simulink model "Doppelpendel_LQG_2014b"  (R2014b)
settings: Solver=ode45  StartTime=0.0  StopTime=15
values from neighbouring files (symbols this model uses):
  Beobachter_Rueckfuehrung = 1    [LoadParameter.m]
  Kalman_Filter = 2    [LoadParameter.m]
  parLQR = LQR_Entwurf(sysd,parLQR)    [A2_5.m]
  Quantisierung = 0    [LoadParameter.m]
undefined symbols (not defined in the file or in its folder): parDP, parKAL
libraries: cstblocks x3
settings Model: CovSFcnEnable=on  Creator=tg  LastModifiedBy=Daniel
settings DataIOCC: SignalLoggingSaveFormat=ModelDataLogs
settings OptimizationCC: ExpressionDepthLimit=2147483647  InitFltsAndDblsToZero=on
settings DebuggingCC: UnderspecifiedInitializationDetection=Classic  MergeDetectMultiDrivingBlocksExec=none  FcnCallInpInsideContextMsg=UseLocalSettings  FrameProcessingCompatibilityMsg=error  StateNameClashWarn=warning
settings SFSimCC: SimParseCustomCode=off
settings GRTTargetCC: CombineOutputUpdateFcns=off  GRTInterface=on

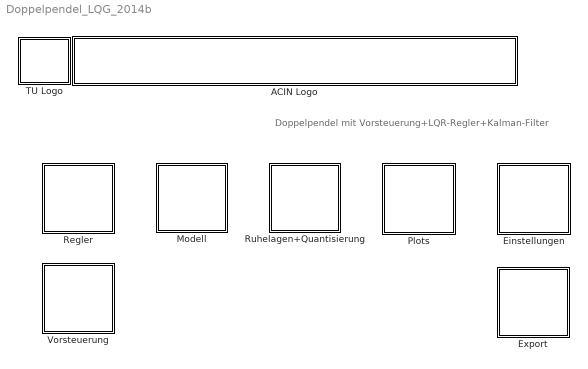
== system Doppelpendel_LQG_2014b ==
  note: Doppelpendel mit Vorsteuerung+LQR-Regler+Kalman-Filter
  ACIN Logo : Subsystem
      mask init:
      | s = get_param(gcb,'UserData');
      mask Display:
      | image(s.logo,[0 0 439 45]);
      | %axis image
  Einstellungen : Subsystem
  Export : Subsystem
  Modell : Subsystem
  Plots : Subsystem
  Regler : Subsystem
  Ruhelagen+Quantisierung : Subsystem
  TU Logo : Subsystem
      mask init:
      | s = get_param(gcb,'UserData');
      mask Display: image(s.logo,[0 0 45 45]);
  Vorsteuerung : Subsystem

== system Doppelpendel_LQG_2014b/ACIN Logo ==

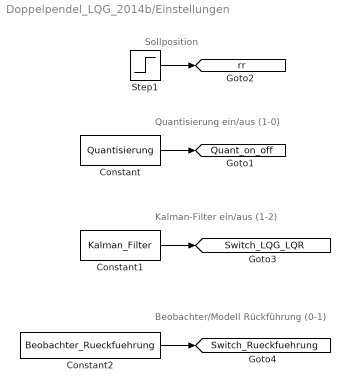
== system Doppelpendel_LQG_2014b/Einstellungen ==
  note: Sollposition
  note: Quantisierung ein/aus (1-0)
  note: Kalman-Filter ein/aus (1-2)
  note: Beobachter/Modell Rückführung (0-1)
  Constant : Constant  Value=Quantisierung
  Constant1 : Constant  Value=Kalman_Filter
  Constant2 : Constant  Value=Beobachter_Rueckfuehrung
  Step1 : Step  After=0.1  SampleTime=parLQR.Ta
  tag scope: Quant_on_off=global, Switch_LQG_LQR=global, Switch_Rueckfuehrung=global, rr=global
  wires:
  Step1/1 -> [rr]
  Constant/1 -> [Quant_on_off]
  Constant1/1 -> [Switch_LQG_LQR]
  Constant2/1 -> [Switch_Rueckfuehrung]

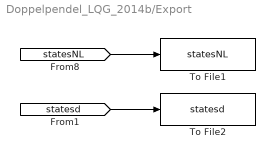
== system Doppelpendel_LQG_2014b/Export ==
  To File1 : ToFile  Filename=statesNL  MatrixName=data  SampleTime=parDP.Ta
  To File2 : ToFile  Filename=statesd  MatrixName=data  SampleTime=parDP.Ta
  wires:
  [statesNL] -> To File1/1
  [statesd] -> To File2/1

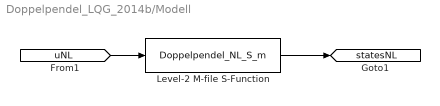
== system Doppelpendel_LQG_2014b/Modell ==
  Level-2 M-file S-Function : M-S-Function  FunctionName=Doppelpendel_NL_S_m  Parameters=parDP.phi10,parDP.omega10,parDP.phi20,parDP.omega20,parDP.s0,parDP.w0,parDP.l1,parDP.l2,parDP.a1,parDP.a2,parDP.m1,parDP.m2,parDP.J1,parDP.J2,parDP.d1,parDP.d2
  tag scope: statesNL=global
  wires:
  [uNL] -> Level-2 M-file S-Function/1
  Level-2 M-file S-Function/1 -> [statesNL]

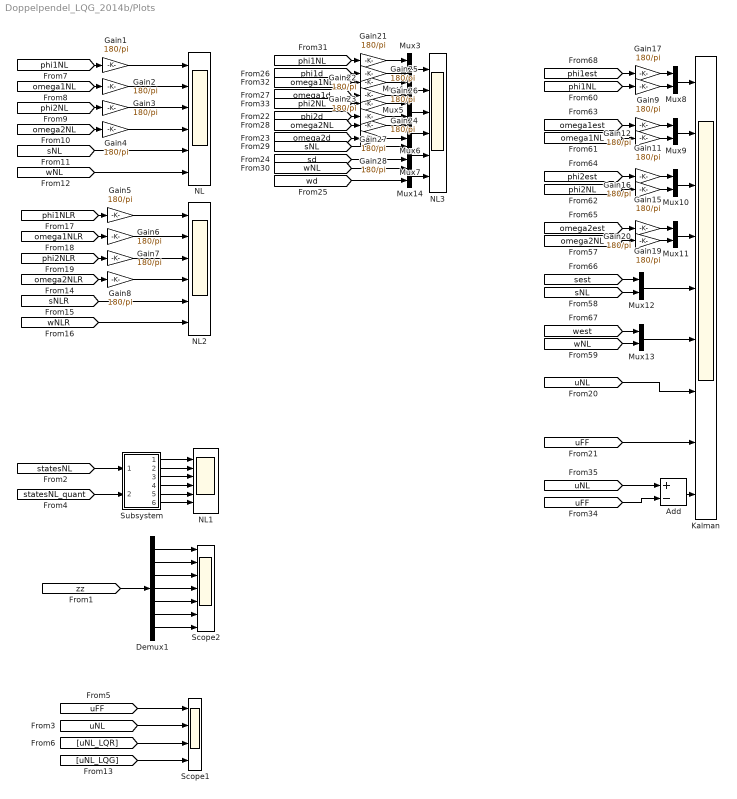
== system Doppelpendel_LQG_2014b/Plots ==
  Add : Sum  Inputs=+-
  Demux1 : Demux  Outputs=7
  Gain{1..9,11..12,15..17,19..28} (24 alike) : Gain  Gain=180/pi
  Kalman : Scope  NumInputPorts=9
      settings: TimeRange=auto  ShowLegends=on  MaxDataPoints=5000  SaveToWorkspace=off  SaveName=ScopeData6  YMin=176.91117~-10.79662~175.59226~-16.92479~-0.25002~-0.32868~-0.36253~-0.36233~-0.00149  YMax=183.0881~10.79663~184.40772~16.91023~0.25002~0.32868~0.36251~0.36233~0.0017  SampleTime=-1
  Mux{3..14} (12 alike) : Mux  Inputs=2
  NL{,1..3} (4 alike) : Scope  NumInputPorts=6
      NL settings: TimeRange=auto  MaxDataPoints=5000  SaveToWorkspace=off  SaveName=ScopeData2  YMin=175.44386~-8.63425~173.59154~-18.09348~-0.06241~-0.43407  YMax=186.73106~14.24878~186.84811~25.58372~0.56166~0.4085  SampleTime=-1
      NL1 settings: TimeRange=auto  MaxDataPoints=5000  SaveToWorkspace=off  YMin=-11.8659~-38.36034~-9.4516~-29.42~-0.73232~-1.57518  YMax=12.13115~31.29264~9.4588~20.36561~0.69417~0.92013  SampleTime=-1
      NL2 settings: TimeRange=auto  MaxDataPoints=5000  SaveToWorkspace=off  SaveName=ScopeData5  YMin=-11.8659~-37.01583~-9.4516~-28.16862~-0.73232~-1.55181  YMax=12.13115~30.14181~9.4588~19.57762~0.69415~0.90614  SampleTime=-1
      NL3 settings: TimeRange=6  MaxDataPoints=5000  SaveToWorkspace=off  SaveName=ScopeData8  YMin=-118.87207~-1672.77009~-161.23535~-3140.598~-141642.31686~-3281468.1161  YMax=19.55566~682.35836~19.81934~939.36059~15738.03521~364607.56846  SampleTime=-1
  Scope1 : Scope  NumInputPorts=4
      settings: TimeRange=6  MaxDataPoints=5000  SaveToWorkspace=off  SaveName=ScopeData4  YMin=-0.36233~-0.36253~-1.00000~-1.00000  YMax=0.36233~0.36251~1.00000~1.00000  SampleTime=-1
  Scope2 : Scope  NumInputPorts=7
      settings: TimeRange=6  MaxDataPoints=5000  SaveToWorkspace=off  SaveName=ScopeData9  YMin=-0.00026~-0.00051~-0.00077~-0.00273~-0.00865~-0.03633~-0.14821  YMax=0.00026~0.00051~0.00077~0.00273~0.00865~0.03633~0.14821  SampleTime=-1
  Subsystem : Subsystem
  wires:
  [omega1NL] -> Gain2/1
  [omega2NL] -> Gain4/1
  [sNL] -> NL/5
  [wNL] -> NL/6
  Gain1/1 -> NL/1
  Gain2/1 -> NL/2
  Gain3/1 -> NL/3
  Gain4/1 -> NL/4
  [phi1NL] -> Gain1/1
  [phi2NL] -> Gain3/1
  [statesNL] -> Subsystem/1(In1)
  [statesNL_quant] -> Subsystem/2(In2)
  Subsystem/1(Out1) -> NL1/1
  Subsystem/2(Out2) -> NL1/2
  Subsystem/3(Out3) -> NL1/3
  Subsystem/4(Out4) -> NL1/4
  Subsystem/5(Out5) -> NL1/5
  Subsystem/6(Out6) -> NL1/6
  [omega1NL] -> Gain22/1
  [omega2NL] -> Gain24/1
  [phi1NL] -> Gain21/1
  [phi2NL] -> Gain23/1
  Mux3/1 -> NL3/1
  Mux4/1 -> NL3/2
  Mux5/1 -> NL3/3
  Mux6/1 -> NL3/4
  Mux7/1 -> NL3/5
  Mux14/1 -> NL3/6
  Gain21/1 -> Mux3/1
  Gain22/1 -> Mux4/1
  Gain23/1 -> Mux5/1
  Gain24/1 -> Mux6/1
  [sNL] -> Mux7/1
  [wNL] -> Mux14/1
  [phi1d] -> Gain25/1
  [omega1d] -> Gain26/1
  [phi2d] -> Gain27/1
  [omega2d] -> Gain28/1
  Gain25/1 -> Mux3/2
  Gain26/1 -> Mux4/2
  Gain27/1 -> Mux5/2
  Gain28/1 -> Mux6/2
  [sd] -> Mux7/2
  [wd] -> Mux14/2
  Demux1/1 -> Scope2/1
  Demux1/2 -> Scope2/2
  Demux1/3 -> Scope2/3
  Demux1/4 -> Scope2/4
  Demux1/5 -> Scope2/5
  Demux1/6 -> Scope2/6
  Demux1/7 -> Scope2/7
  [zz] -> Demux1/1
  Mux13/1 -> Kalman/6
  Mux12/1 -> Kalman/5
  Mux11/1 -> Kalman/4
  [omega1NL] -> Gain12/1
  [omega2NL] -> Gain20/1
  [phi1NL] -> Gain9/1
  [phi2NL] -> Gain16/1
  [sest] -> Mux12/1
  [west] -> Mux13/1
  [sNL] -> Mux12/2
  [wNL] -> Mux13/2
  Gain9/1 -> Mux8/2
  Gain17/1 -> Mux8/1
  [phi1est] -> Gain17/1
  Mux8/1 -> Kalman/1
  Gain12/1 -> Mux9/2
  Gain11/1 -> Mux9/1
  Mux9/1 -> Kalman/2
  [omega1est] -> Gain11/1
  Gain16/1 -> Mux10/2
  Gain15/1 -> Mux10/1
  [phi2est] -> Gain15/1
  Mux10/1 -> Kalman/3
  Gain20/1 -> Mux11/2
  Gain19/1 -> Mux11/1
  [omega2est] -> Gain19/1
  [uFF] -> Scope1/1
  [uNL] -> Scope1/2
  [uNL_LQR] -> Scope1/3
  [uNL_LQG] -> Scope1/4
  [omega1NLR] -> Gain6/1
  [omega2NLR] -> Gain8/1
  [sNLR] -> NL2/5
  [wNLR] -> NL2/6
  Gain5/1 -> NL2/1
  Gain6/1 -> NL2/2
  Gain7/1 -> NL2/3
  Gain8/1 -> NL2/4
  [phi1NLR] -> Gain5/1
  [phi2NLR] -> Gain7/1
  [uNL] -> Kalman/7
  [uFF] -> Kalman/8
  Add/1 -> Kalman/9
  [uNL] -> Add/1
  [uFF] -> Add/2

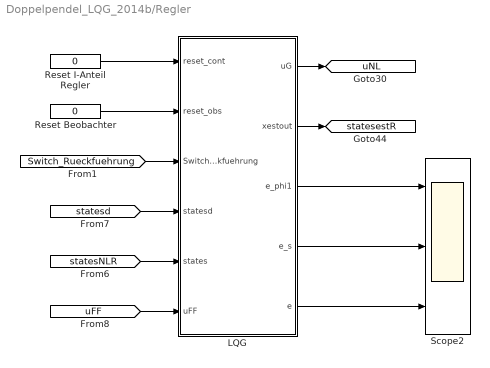
== system Doppelpendel_LQG_2014b/Regler ==
  LQG : MATLAB Function  TreatAsAtomicUnit=on
      settings: PermitHierarchicalResolution=ParametersOnly
  Reset Beobachter : Constant  Value=0
  Reset I-Anteil Regler : Constant  Value=0
  Scope2 : Scope  NumInputPorts=3
      settings: TimeRange=auto  MaxDataPoints=5000  SaveToWorkspace=off  SaveName=ScopeData  YMin=-0.00033~-0.00072~-30.14504  YMax=0.00036~0.00074~27.50332  SampleTime=-1
  tag scope: statesestR=global, uNL=global
  wires:
  LQG/3(e_phi1) -> Scope2/1
  LQG/4(e_s) -> Scope2/2
  LQG/5(e) -> Scope2/3
  [statesNLR] -> LQG/5(states)
  LQG/2(xestout) -> [statesestR]
  [statesd] -> LQG/4(statesd)
  [uFF] -> LQG/6(uFF)
  LQG/1(uG) -> [uNL]
  Reset Beobachter/1 -> LQG/2(reset_obs)
  Reset I-Anteil Regler/1 -> LQG/1(reset_cont)
  [Switch_Rueckfuehrung] -> LQG/3(Switch_Rueckfuehrung)

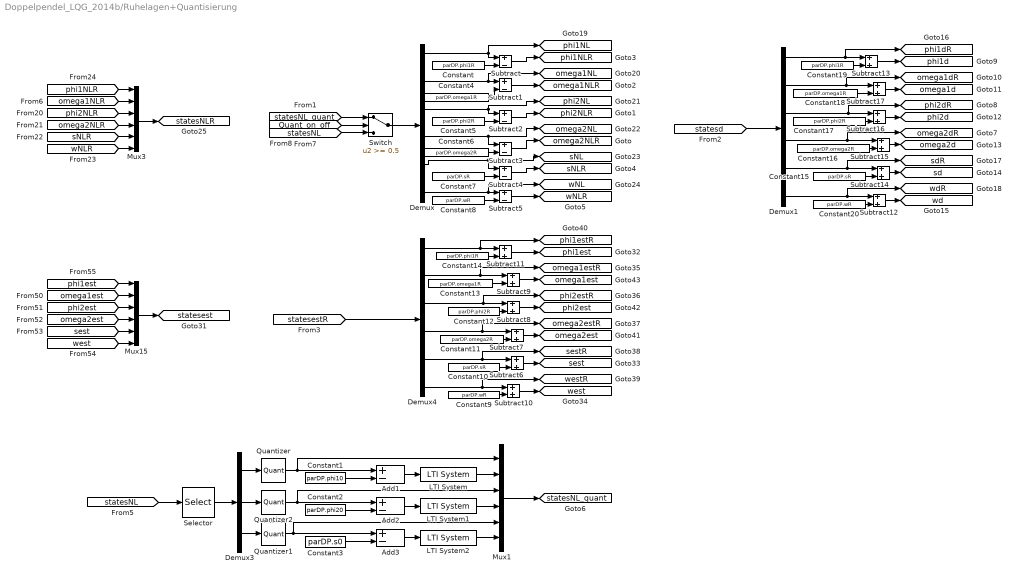
== system Doppelpendel_LQG_2014b/Ruhelagen+Quantisierung ==
  Add1 : Sum  Inputs=+-
  Add2 : Sum  Inputs=+-
  Add3 : Sum  Inputs=+-
  Constant : Constant  Value=parDP.phi1R
  Constant1 : Constant  Value=parDP.phi10
  Constant10 : Constant  Value=parDP.sR
  Constant11 : Constant  Value=parDP.omega2R
  Constant12 : Constant  Value=parDP.phi2R
  Constant13 : Constant  Value=parDP.omega1R
  Constant14 : Constant  Value=parDP.phi1R
  Constant15 : Constant  Value=parDP.sR
  Constant16 : Constant  Value=parDP.omega2R
  Constant17 : Constant  Value=parDP.phi2R
  Constant18 : Constant  Value=parDP.omega1R
  Constant19 : Constant  Value=parDP.phi1R
  Constant2 : Constant  Value=parDP.phi20
  Constant20 : Constant  Value=parDP.wR
  Constant3 : Constant  Value=parDP.s0
  Constant4 : Constant  Value=parDP.omega1R
  Constant5 : Constant  Value=parDP.phi2R
  Constant6 : Constant  Value=parDP.omega2R
  Constant7 : Constant  Value=parDP.sR
  Constant8 : Constant  Value=parDP.wR
  Constant9 : Constant  Value=parDP.wR
  Demux : Demux  Outputs=6
  Demux1 : Demux  Outputs=6
  Demux3 : Demux  Outputs=3
  Demux4 : Demux  Outputs=6
  LTI System : cstblocks/LTI System  sys=Fd_diff  IC=[]
  LTI System1 : cstblocks/LTI System  sys=Fd_diff  IC=[]
  LTI System2 : cstblocks/LTI System  sys=Fd_diff  IC=[]
  Mux1 : Mux  Inputs=6
  Mux15 : Mux  Inputs=6
  Mux3 : Mux  Inputs=6
  Quantizer : Quantizer  QuantizationInterval=Phiquantisierung  SampleTime=parLQR.Ta
  Quantizer1 : Quantizer  QuantizationInterval=Wegquantisierung  SampleTime=parLQR.Ta
  Quantizer2 : Quantizer  QuantizationInterval=Phiquantisierung  SampleTime=parLQR.Ta
  Selector : Selector  InputPortWidth=6  IndexOptions=Index vector (dialog)  Indices=[1 3 5]  OutputSizes=1
  Subtract{,1..5} (6 alike) : Sum  Inputs=+-
  Subtract{6..17} (12 alike) : Sum
  Switch : Switch  Threshold=0.5
  tag scope: omega1NL=global, omega1NLR=global, omega1d=global, omega1dR=global, omega1est=global, omega1estR=global, omega2NL=global, omega2NLR=global, omega2d=global, omega2dR=global, omega2est=global, omega2estR=global, phi1NL=global, phi1NLR=global, phi1d=global, phi1dR=global, phi1est=global, phi1estR=global, phi2NL=global, phi2NLR=global, phi2d=global, phi2dR=global, phi2est=global, phi2estR=global, sNL=global, sNLR=global, sd=global, sdR=global, sest=global, sestR=global, statesNLR=global, statesNL_quant=global, statesest=global, wNL=global, wNLR=global, wd=global, wdR=global, west=global, westR=global
  wires:
  [phi1NLR] -> Mux3/1
  [omega1NLR] -> Mux3/2
  [phi2NLR] -> Mux3/3
  [omega2NLR] -> Mux3/4
  [sNLR] -> Mux3/5
  [wNLR] -> Mux3/6
  Mux3/1 -> [statesNLR]
  [phi1est] -> Mux15/1
  [omega1est] -> Mux15/2
  [phi2est] -> Mux15/3
  [omega2est] -> Mux15/4
  [sest] -> Mux15/5
  [west] -> Mux15/6
  Mux15/1 -> [statesest]
  [statesNL] -> Selector/1
  Selector/1 -> Demux3/1
  Demux3/2 -> Quantizer2/1
  Demux3/1 -> Quantizer/1
  Demux3/3 -> Quantizer1/1
  Mux1/1 -> [statesNL_quant]
  LTI System/1 -> Mux1/2
  LTI System2/1 -> Mux1/6
  LTI System1/1 -> Mux1/4
  Add1/1 -> LTI System/1
  Add2/1 -> LTI System1/1
  Add3/1 -> LTI System2/1
  Constant1/1 -> Add1/2
  Constant2/1 -> Add2/2
  Constant3/1 -> Add3/2
  Quantizer1/1 -> Add3/1, Mux1/5
  Quantizer2/1 -> Add2/1, Mux1/3
  Quantizer/1 -> Add1/1, Mux1/1
  [statesestR] -> Demux4/1
  Switch/1 -> Demux/1
  [Quant_on_off] -> Switch/2
  [statesNL_quant] -> Switch/1
  [statesNL] -> Switch/3
  [statesd] -> Demux1/1
  Constant/1 -> Subtract/2
  Subtract/1 -> [phi1NLR]
  Demux/1 -> [phi1NL], Subtract/1
  Constant4/1 -> Subtract1/2
  Demux/2 -> [omega1NL], Subtract1/1
  Subtract1/1 -> [omega1NLR]
  Constant5/1 -> Subtract2/2
  Subtract2/1 -> [phi2NLR]
  Demux/3 -> [phi2NL], Subtract2/1
  Constant6/1 -> Subtract3/2
  Subtract3/1 -> [omega2NLR]
  Demux/4 -> [omega2NL], Subtract3/1
  Constant7/1 -> Subtract4/2
  Subtract4/1 -> [sNLR]
  Demux/5 -> Subtract4/1, [sNL]
  Constant8/1 -> Subtract5/2
  Subtract5/1 -> [wNLR]
  Demux/6 -> [wNL], Subtract5/1
  Demux4/2 -> Subtract9/1, [omega1estR]
  Demux4/3 -> [phi2estR], Subtract8/1
  Demux4/4 -> [omega2estR], Subtract7/1
  Demux4/6 -> Subtract10/1, [westR]
  Subtract11/1 -> [phi1est]
  Subtract9/1 -> [omega1est]
  Subtract8/1 -> [phi2est]
  Subtract7/1 -> [omega2est]
  Subtract6/1 -> [sest]
  Subtract10/1 -> [west]
  Demux4/1 -> Subtract11/1, [phi1estR]
  Demux4/5 -> [sestR], Subtract6/1
  Constant9/1 -> Subtract10/2
  Constant10/1 -> Subtract6/2
  Constant11/1 -> Subtract7/2
  Constant12/1 -> Subtract8/2
  Constant13/1 -> Subtract9/2
  Constant14/1 -> Subtract11/2
  Demux1/2 -> [omega1dR], Subtract17/1
  Demux1/3 -> [phi2dR], Subtract16/1
  Demux1/4 -> [omega2dR], Subtract15/1
  Demux1/6 -> [wdR], Subtract12/1
  Subtract13/1 -> [phi1d]
  Subtract17/1 -> [omega1d]
  Subtract16/1 -> [phi2d]
  Subtract15/1 -> [omega2d]
  Subtract14/1 -> [sd]
  Subtract12/1 -> [wd]
  Demux1/1 -> [phi1dR], Subtract13/1
  Demux1/5 -> [sdR], Subtract14/1
  Constant20/1 -> Subtract12/2
  Constant15/1 -> Subtract14/2
  Constant16/1 -> Subtract15/2
  Constant17/1 -> Subtract16/2
  Constant18/1 -> Subtract17/2
  Constant19/1 -> Subtract13/2

== system Doppelpendel_LQG_2014b/TU Logo ==

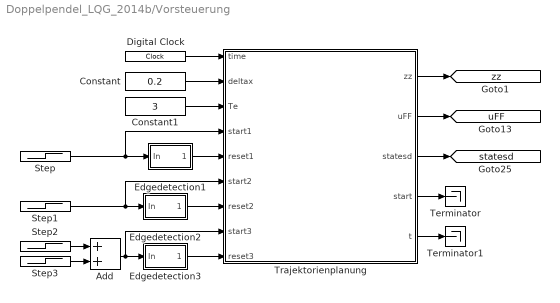
== system Doppelpendel_LQG_2014b/Vorsteuerung ==
  Add : Sum
  Constant : Constant  Value=0.2
  Constant1 : Constant  Value=3
  Digital Clock : DigitalClock  SampleTime=parLQR.Ta
  Edgedetection1 : Subsystem
  Edgedetection2 : Subsystem
  Edgedetection3 : Subsystem
  Step : Step  Time=2  SampleTime=0
  Step1 : Step  Time=6  SampleTime=0
  Step2 : Step  Time=14  After=-1  SampleTime=0
  Step3 : Step  Time=10  SampleTime=0
  Terminator : Terminator
  Terminator1 : Terminator
  Trajektorienplanung : MATLAB Function  TreatAsAtomicUnit=on
      settings: PermitHierarchicalResolution=ParametersOnly
  tag scope: statesd=global, uFF=global, zz=global
  wires:
  Trajektorienplanung/1(zz) -> [zz]
  Trajektorienplanung/5(t) -> Terminator1/1
  Trajektorienplanung/4(start) -> Terminator/1
  Step3/1 -> Add/2
  Step2/1 -> Add/1
  Edgedetection3/1(Out1) -> Trajektorienplanung/9(reset3)
  Step1/1 -> Edgedetection2/1(In), Trajektorienplanung/6(start2)
  Edgedetection2/1(Out1) -> Trajektorienplanung/7(reset2)
  Edgedetection1/1(Out1) -> Trajektorienplanung/5(reset1)
  Digital Clock/1 -> Trajektorienplanung/1(time)
  Trajektorienplanung/3(statesd) -> [statesd]
  Step/1 -> Edgedetection1/1(In), Trajektorienplanung/4(start1)
  Trajektorienplanung/2(uFF) -> [uFF]
  Constant/1 -> Trajektorienplanung/2(deltax)
  Constant1/1 -> Trajektorienplanung/3(Te)
  Add/1 -> Edgedetection3/1(In), Trajektorienplanung/8(start3)

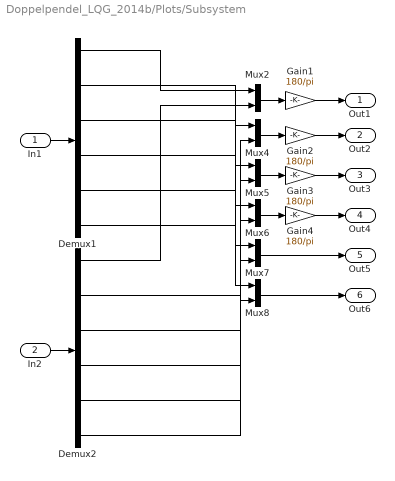
== system Doppelpendel_LQG_2014b/Plots/Subsystem ==
  In1 : Inport
  In2 : Inport  Port=2
  Demux1 : Demux  Outputs=6
  Demux2 : Demux  Outputs=6
  Gain{1..4} (4 alike) : Gain  Gain=180/pi
  Mux{2,4..8} (6 alike) : Mux  Inputs=2
  Out1 : Outport
  Out2 : Outport  Port=2
  Out3 : Outport  Port=3
  Out4 : Outport  Port=4
  Out5 : Outport  Port=5
  Out6 : Outport  Port=6
  wires:
  Demux1/1 -> Mux2/1
  Demux2/1 -> Mux2/2
  Demux2/2 -> Mux4/2
  Demux2/3 -> Mux5/2
  Demux2/4 -> Mux6/2
  Demux2/5 -> Mux7/2
  Demux2/6 -> Mux8/2
  Demux1/6 -> Mux8/1
  Demux1/5 -> Mux7/1
  Demux1/2 -> Mux4/1
  Demux1/3 -> Mux5/1
  Demux1/4 -> Mux6/1
  Mux2/1 -> Gain1/1
  Mux4/1 -> Gain2/1
  In1/1 -> Demux1/1
  Mux5/1 -> Gain3/1
  Mux6/1 -> Gain4/1
  Mux7/1 -> Out5/1
  Mux8/1 -> Out6/1
  In2/1 -> Demux2/1
  Gain1/1 -> Out1/1
  Gain2/1 -> Out2/1
  Gain3/1 -> Out3/1
  Gain4/1 -> Out4/1

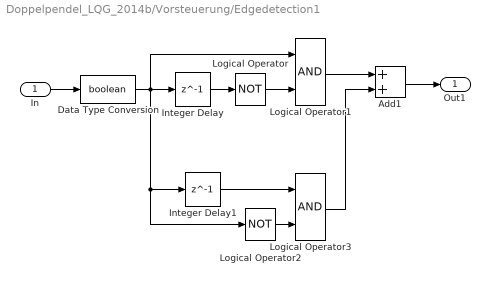
== system Doppelpendel_LQG_2014b/Vorsteuerung/Edgedetection1 ==
  In : Inport
  Add1 : Sum
  Data Type Conversion : DataTypeConversion  OutDataTypeStr=boolean  SaturateOnIntegerOverflow=on  RndMeth=Zero
  Integer Delay : Delay  DelayLength=1  InputProcessing=Inherited  SampleTime=parLQR.Ta
  Integer Delay1 : Delay  DelayLength=1  InputProcessing=Inherited  SampleTime=parLQR.Ta
  Logical Operator : Logic  Operator=NOT  Inputs=1
  Logical Operator1 : Logic
  Logical Operator2 : Logic  Operator=NOT  Inputs=1
  Logical Operator3 : Logic
  Out1 : Outport
  wires:
  In/1 -> Data Type Conversion/1
  Integer Delay/1 -> Logical Operator/1
  Data Type Conversion/1 -> Logical Operator1/1, Integer Delay/1, Integer Delay1/1, Logical Operator2/1
  Logical Operator/1 -> Logical Operator1/2
  Logical Operator2/1 -> Logical Operator3/2
  Integer Delay1/1 -> Logical Operator3/1
  Logical Operator1/1 -> Add1/1
  Logical Operator3/1 -> Add1/2
  Add1/1 -> Out1/1

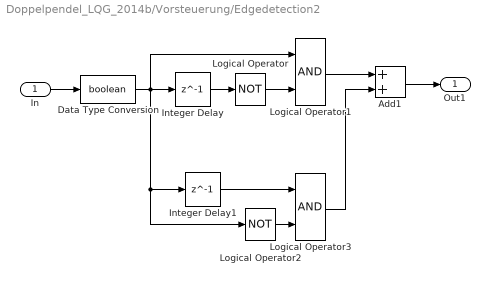
== system Doppelpendel_LQG_2014b/Vorsteuerung/Edgedetection2 ==
  In : Inport
  Add1 : Sum
  Data Type Conversion : DataTypeConversion  OutDataTypeStr=boolean  SaturateOnIntegerOverflow=on  RndMeth=Zero
  Integer Delay : Delay  DelayLength=1  InputProcessing=Inherited  SampleTime=parLQR.Ta
  Integer Delay1 : Delay  DelayLength=1  InputProcessing=Inherited  SampleTime=parLQR.Ta
  Logical Operator : Logic  Operator=NOT  Inputs=1
  Logical Operator1 : Logic
  Logical Operator2 : Logic  Operator=NOT  Inputs=1
  Logical Operator3 : Logic
  Out1 : Outport
  wires:
  Add1/1 -> Out1/1
  Logical Operator3/1 -> Add1/2
  Logical Operator1/1 -> Add1/1
  Integer Delay1/1 -> Logical Operator3/1
  Logical Operator2/1 -> Logical Operator3/2
  Logical Operator/1 -> Logical Operator1/2
  Data Type Conversion/1 -> Logical Operator2/1, Integer Delay1/1, Integer Delay/1, Logical Operator1/1
  Integer Delay/1 -> Logical Operator/1
  In/1 -> Data Type Conversion/1

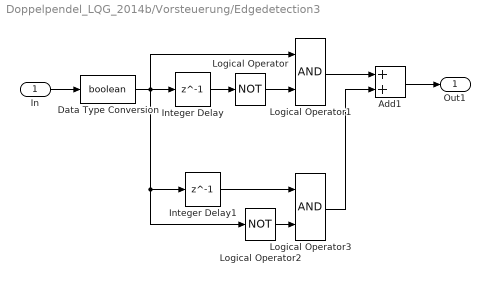
== system Doppelpendel_LQG_2014b/Vorsteuerung/Edgedetection3 ==
  In : Inport
  Add1 : Sum
  Data Type Conversion : DataTypeConversion  OutDataTypeStr=boolean  SaturateOnIntegerOverflow=on  RndMeth=Zero
  Integer Delay : Delay  DelayLength=1  InputProcessing=Inherited  SampleTime=parLQR.Ta
  Integer Delay1 : Delay  DelayLength=1  InputProcessing=Inherited  SampleTime=parLQR.Ta
  Logical Operator : Logic  Operator=NOT  Inputs=1
  Logical Operator1 : Logic
  Logical Operator2 : Logic  Operator=NOT  Inputs=1
  Logical Operator3 : Logic
  Out1 : Outport
  wires:
  In/1 -> Data Type Conversion/1
  Integer Delay/1 -> Logical Operator/1
  Data Type Conversion/1 -> Logical Operator1/1, Integer Delay/1, Integer Delay1/1, Logical Operator2/1
  Logical Operator/1 -> Logical Operator1/2
  Logical Operator2/1 -> Logical Operator3/2
  Integer Delay1/1 -> Logical Operator3/1
  Logical Operator1/1 -> Add1/1
  Logical Operator3/1 -> Add1/2
  Add1/1 -> Out1/1

== matlab function Doppelpendel_LQG_2014b/Regler/LQG ==
  settings: updateMethod=DISCRETE  sampleTime=parLQR.Ta
  data: reset_cont input; reset_obs input; Switch_Rueckfuehrung input; statesd input; states input; uFF input; uG output; parLQR parameter; xestout output; e_phi1 output; e_s output; parKAL parameter; e output
function [uG,xestout,e_phi1,e_s,e]  = LQG(reset_cont,reset_obs,Switch_Rueckfuehrung,statesd,states,uFF,parLQR,parKAL)

%Anfangsbedinungen
persistent eI
if isempty(eI) eI = double(0); end

persistent phi1est
if isempty(phi1est)phi1est = 0; end
persistent omega1est
if isempty(omega1est)omega1est = 0; end
persistent phi2est
if isempty(phi2est)phi2est = 0; end
persistent omega2est
if isempty(omega2est)omega2est = 0; end
persistent sest
if isempty(sest)sest = 0; end
persistent west
if isempty(west)west = 0; end

%Ausgang
xestout=[phi1est,omega1est,phi2est,omega2est,sest,west]';

%Beobachterrückführung ein/aus
if (Switch_Rueckfuehrung)
    xest=xestout;
else
    xest=states;
end
%%%%%%%%%%%%%%%%%%%%%%%%%%%%%%%%%%%%%%%%%%%%%%%%%%%%%%%%%%%%%%%%%%%%%%%%%%%
%LQR-Regler
%%%%%%%%%%%%%%%%%%%%%%%%%%%%%%%%%%%%%%%%%%%%%%%%%%%%%%%%%%%%%%%%%%%%%%%%%%%

% Folgendes hier bitte ausführen:
% 1.) PI-Zustandsregler einfügen
% 2.) if (reset_cont==1) xI=0 end

if(reset_cont==1)
   eI=0; 
end

if(Switch_Rueckfuehrung)
    uFB = [parLQR.kx parLQR.kI]*[xest-statesd;eI];
    eI = eI+(statesd(5)-xest(5));
else
    uFB = [parLQR.kx parLQR.kI]*[states-statesd;eI];
    eI = eI+(statesd(5)-states(5));
end   
%Gesamtrückführung
uG=uFF+uFB;

%%%%%%%%%%%%%%%%%%%%%%%%%%%%%%%%%%%%%%%%%%%%%%%%%%%%%%%%%%%%%%%%%%%%%%%%%%%
%Kalman-Filter
%%%%%%%%%%%%%%%%%%%%%%%%%%%%%%%%%%%%%%%%%%%%%%%%%%%%%%%%%%%%%%%%%%%%%%%%%%%

% Folgendes hier bitte ausführen:
% 1.) Kalman-Filter einfügen
% 2.) if (reset_obs==1) xestout=[0,0,0,0,0,0]' end

if(reset_obs==1)
    xestout=[0,0,0,0,0,0]'; 
end

% Formel 2.79
xest= parKAL.Asysd*xest+parKAL.bsysd*uG+parKAL.KK*([states(1);states(5)]-[xest(1);xest(5)]);

 phi1est=xest(1);
 omega1est=xest(2);
 phi2est=xest(3);
 omega2est=xest(4);
 sest=xest(5);
 west=xest(6);

e_phi1=states(1)-phi1est;
e_s=states(5)-sest;
e=eI;

== matlab function Doppelpendel_LQG_2014b/Vorsteuerung/Trajektorienplanung ==
  settings: updateMethod=DISCRETE  sampleTime=parLQR.Ta
  data: time input; deltax input; Te input; zz output; parFF parameter; uFF output; statesd output; start1 input; reset1 input; start2 input; start output; reset2 input; t output; start3 input; reset3 input
% Trajektorienplanung zum Versetzten des Doppelpendels
function [zz,uFF,statesd,start,t] = Trajektorienplanung(time,deltax,Te,parFF,start1,reset1,start2,reset2,start3,reset3)

persistent tstart
if isempty(tstart) tstart = double(0); end
persistent x0
if isempty(x0) x0 = double(0); end
persistent xT
if isempty(xT) xT = double(deltax); end


if reset1>0.5 || reset2>0.5 || reset3>0.5
    
    tstart = time;

end
%Zeit ab tstart
t = time - tstart;


if  start1>0.5 
    
    start = 1;
    
    if start2<0.5
        
        x0=0;
        xT=deltax; 
        
    else
        
        if start3<0.5
        
            x0=deltax;
            xT=-deltax; 
        
        else
    
            %Anfangs- und Endwert
            x0=-deltax;
            xT=deltax;
            
        end

    end
    
else
    
    start = 0;
    
end

% Folgendes hier bitte ausführen:
% 1.) Umrechnung auf Anfangs- und Endwert des Flachen Ausgangs
% 2.) Funktion Trajektorie() ergänzen
% 3.) Vorsteuerungsberechnung uFF ergänzen
% 4.) Sollzustandsverlauf statesd ergänzen

%Umrechnung auf Anfangs- und Endwert des Flachen Ausgangs
xi0 = parFF.VVinv\[0;0;0;0;x0;0];
xiT = parFF.VVinv\[0;0;0;0;xT;0];

z0 = xi0(1);
zT = xiT(1);


zz = Trajektorie(start,t,Te,z0,zT,parFF);
%zz=[z,zdot,z2dot,z3dot,z4dot,z5dot,z6dot];

%Vorsteuerung
uFF = parFF.aa*zz';
%Sollzustandsverlauf
statesd = parFF.VVinv*zz(1:end-1)';
end

%%%%%%%%%%%%%%%%%%%%%%%%%%%%%%%%%%%%%%%%%%%%%%%%%%%%%%%%%%%%%%%%%%%%%%%%%%    
function [zz] = Trajektorie(start,t,Te,z0,zT,parFF)
    beta7 = parFF.beta7;
    beta8 = parFF.beta8;
    beta9 = parFF.beta9;
    beta10 = parFF.beta10;
    beta11 = parFF.beta11;
    beta12 = parFF.beta12;
    beta13 = parFF.beta13;
    T = Te;
    
    if start<0.5

        z     = z0; 
        zdot  = 0; 
        z2dot = 0; 
        z3dot = 0; 
        z4dot = 0; 
        z5dot = 0; 
        z6dot = 0; 

    elseif start>0.5 && t<Te

        % Folgendes hier bitte ausführen:
        % 1.) Berechnung der Solltrajektorie
        z = z0 + (zT - z0) * (beta7 * t .^ 7 / T .^ 7 + beta8 * t .^ 8 / T .^ 8 + beta9 * t .^ 9 / T .^ 9 + beta10 * t .^ 10 / T .^ 10 + beta11 * t .^ 11 / T .^ 11 + beta12 * t .^ 12 / T .^ 12 + beta13 * t .^ 13 / T .^ 13);
        zdot = (zT - z0) * (7 * beta7 * t .^ 6 / T .^ 7 + 8 * beta8 * t .^ 7 / T .^ 8 + 9 * beta9 * t .^ 8 / T .^ 9 + 10 * beta10 * t .^ 9 / T .^ 10 + 11 * beta11 * t .^ 10 / T .^ 11 + 12 * beta12 * t .^ 11 / T .^ 12 + 13 * beta13 * t .^ 12 / T .^ 13);
        z2dot = (zT - z0) * (42 * beta7 * t .^ 5 / T .^ 7 + 56 * beta8 * t .^ 6 / T .^ 8 + 72 * beta9 * t .^ 7 / T .^ 9 + 90 * beta10 * t .^ 8 / T .^ 10 + 110 * beta11 * t .^ 9 / T .^ 11 + 132 * beta12 * t .^ 10 / T .^ 12 + 156 * beta13 * t .^ 11 / T .^ 13);
        z3dot = (zT - z0) * (210 * beta7 * t .^ 4 / T .^ 7 + 336 * beta8 * t .^ 5 / T .^ 8 + 504 * beta9 * t .^ 6 / T .^ 9 + 720 * beta10 * t .^ 7 / T .^ 10 + 990 * beta11 * t .^ 8 / T .^ 11 + 1320 * beta12 * t .^ 9 / T .^ 12 + 1716 * beta13 * t .^ 10 / T .^ 13);
        z4dot = (zT - z0) * (840 * beta7 * t .^ 3 / T .^ 7 + 1680 * beta8 * t .^ 4 / T .^ 8 + 3024 * beta9 * t .^ 5 / T .^ 9 + 5040 * beta10 * t .^ 6 / T .^ 10 + 7920 * beta11 * t .^ 7 / T .^ 11 + 11880 * beta12 * t .^ 8 / T .^ 12 + 17160 * beta13 * t .^ 9 / T .^ 13);
        z5dot = (zT - z0) * (2520 * beta7 * t .^ 2 / T .^ 7 + 6720 * beta8 * t .^ 3 / T .^ 8 + 15120 * beta9 * t .^ 4 / T .^ 9 + 30240 * beta10 * t .^ 5 / T .^ 10 + 55440 * beta11 * t .^ 6 / T .^ 11 + 95040 * beta12 * t .^ 7 / T .^ 12 + 154440 * beta13 * t .^ 8 / T .^ 13);
        z6dot = (zT - z0) * (5040 * beta7 * t / T .^ 7 + 20160 * beta8 * t .^ 2 / T .^ 8 + 60480 * beta9 * t .^ 3 / T .^ 9 + 151200 * beta10 * t .^ 4 / T .^ 10 + 332640 * beta11 * t .^ 5 / T .^ 11 + 665280 * beta12 * t .^ 6 / T .^ 12 + 1235520 * beta13 * t .^ 7 / T .^ 13);


    else

        z     = zT; 
        zdot  = 0; 
        z2dot = 0; 
        z3dot = 0; 
        z4dot = 0; 
        z5dot = 0; 
        z6dot = 0; 

    end

    zz=[z,zdot,z2dot,z3dot,z4dot,z5dot,z6dot];

end
